simulink model "InductionMotorDrive"  (R2024a)
settings: Solver=FixedStepDiscrete  StartTime=0.0  StopTime=3  RelTol=1e-3  EnableMultiTasking=on
PreLoadFcn:
  | Ts=2e-6;
libraries: spsStairGeneratorLib x3, spsACVoltageSourceLib x1, electricdrivelib x1, sps_lib x1
settings Model: Creator=The MathWorks, Inc.
settings SolverCC: AlgebraicLoopSolver=TrustRegion
settings DataIOCC: SaveFormat=Array  SaveOutput=off  SignalLogging=off  SaveTime=off  ReturnWorkspaceOutputs=off
settings OptimizationCC: LifeSpan=inf
settings DebuggingCC: UnconnectedInputMsg=warning  UnconnectedOutputMsg=warning  UnconnectedLineMsg=warning  SFUnexpectedBacktrackingDiag=warning  SFNoUnconditionalDefaultTransitionDiag=warning  SFExecutionAtInitializationDiag=none  ArithmeticOperatorsInVariantConditions=warning
settings HardwareCC: ProdBitPerSizeT=32  ProdBitPerPtrDiffT=32  ProdWordSize=32  ProdHWDeviceType=Specified
settings ModelReferenceCC: EnableRefExpFcnMdlSchedulingChecks=on
settings SFSimCC: SimUseLocalCustomCode=off  CustomCodeUndefinedFunction=UseInterfaceOnly
settings RTWCC: RTWUseLocalCustomCode=off  GPUComputeCapability=3.5
settings CodeAppCC: StateflowObjectComments=on
settings GRTTargetCC: TargetLangStandard=C89/C90 (ANSI)
settings ConfigComp: CovMetricSettings=dw  CovSaveCumulativeToWorkspaceVar=on  CovSaveSingleToWorkspaceVar=on  CovExternalEMLEnable=off
settings SimscapeCC: SimscapeNormalizeSystem=off  SimscapeNominalValues={1, 'bar'; 1, 'cm^3/s'; 1, 'bar*kg/s'; 1, 'kJ/kg'; 1, 'kW'; }

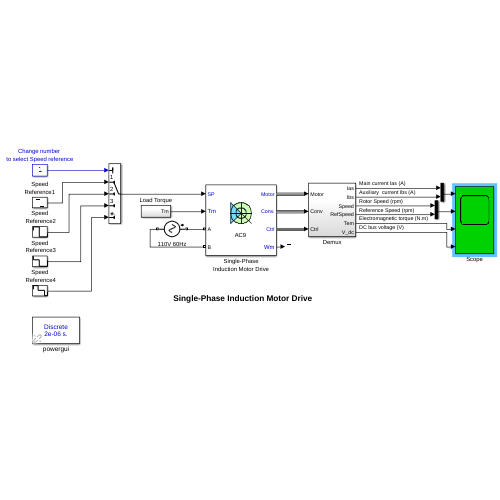
[thumbnail: Simulink's stored preview of the top-level diagram]
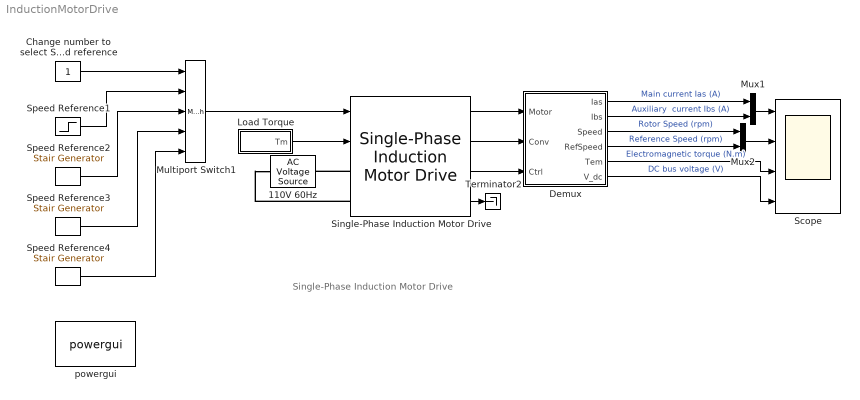
== system InductionMotorDrive ==
  note: Single-Phase Induction Motor Drive
  110V 60Hz : spsACVoltageSourceLib/AC Voltage Source  Amplitude=110*sqrt(2)  Phase=0  Frequency=60  SampleTime=0  Measurements=None  BusType=swing  Pref=10e3  Qref=0  Qmin=-inf  Qmax=+inf
  Change number to select Speed reference : Constant
  Demux : Subsystem
  Load Torque : Subsystem
  Multiport Switch1 : MultiPortSwitch  Inputs=4  InputSameDT=off
  Mux1 : Mux  Inputs=2
  Mux2 : Mux  Inputs=2
  Scope : Scope  NumInputPorts=4
  Single-Phase Induction Motor Drive : electricdrivelib/AC drives/Single-Phase Induction Motor Drive  Pn=0.25*746  Vn=110  fn=60  Rs=2.02  Lls=7.4e-3  Lms=0.1772  Ra=7.14  Lla=8.5e-3  k=1.18  Rr=4.12  Llr=5.6e-3  J=0.0146  Friction=0  p=2  InitialSpeed=0  Rsnubber1=10e3  Csnubber1=20e-9  Ron1=1e-3  Vf1=0.8  cap_bus=39e-4  Rbrake=8  fbrake=4000  activationVoltage=310  shutdownVoltage=300  deviceType=IGBT / Diodes  Ron2=1e-3  Vf2=0  Vfd=0  Rsnubber2=5000  Csnubber2=inf  regulationType=Speed regulation  Tsc=7*20e-6  fc_sc=1000  Acc=1800  Dec=-1800  kp_sc=1  ki_sc=10  Tmin=-4  Tmax=4  in_flux=0.3  nf=0.3  controllerType=FOC  h=0.5  T_bw=0.1  F_bw=0.002  freq_max=20000  Tvect=20e-6  baseSampleTime=2e-06  outputBusMode=Multiple output buses  busLabels=off  MechanicalLoad=Torque Tm  driveType=AC9
  Speed Reference2 : spsStairGeneratorLib/Stair Generator  t=[0 1 1.5 2.2]  e=[500 1000 -500 0]  Ts=Ts
  Speed Reference3 : spsStairGeneratorLib/Stair Generator  t=[0 1 1.5 2.2]  e=[1250 600 -500 500]  Ts=Ts
  Speed Reference4 : spsStairGeneratorLib/Stair Generator  t=[0 1 1.5 2.2 2.5]  e=[500 1000 300 -500 0]  Ts=Ts
  Speed Reference1 : Step  Before=1500  After=750  SampleTime=0
  Terminator2 : Terminator
  powergui : sps_lib/powergui  Priority=2  SimulationMode=Discrete  SampleTime=Ts  frequency=60  Iterations=50  frequencyindice=60  Pbase=100e6  ErrMax=1e-4  UnitsV=kV  UnitsW=MW  buscounter=0  FunctionMessages=off  echomessages=off  EnableUseOfTLC=off  CurrentSourceSwitches=off  DisableSnubberDevices=off  DisableRonSwitches=off  DisableVfSwitches=off  DisplayEquations=off  AutomaticDiscreteSolvers=off  SolverType=Tustin/Backward Euler (TBE)  Interpol=off  ExternalGateDelay=off  methode=off  Ts=0  x0status=blocks  SPID=off  SwTol=0  HookPort=off  NonlinearTolerance=0  nMaxIteration=15  ContinueOnMaxIteration=off  RestoreLinks=warning  ResistiveCurrentMeasurement=off  Frange=[0:2:500]  Ylog=off  Xlog=on  ShowGrid=off  save=off  variable=ZData  structure=0  ZoomFFT=on  StartTime=0.0  cycles=1  DisplayStyle=1  fundamental=60  FreqAxis=off  MaxFrequency=1000  frequencyindicesteady=1  RmsSteady=1  display=off
  wires:
  Single-Phase Induction Motor Drive/4 -> Terminator2/1
  Load Torque/1(Tm) -> Single-Phase Induction Motor Drive/2
  Speed Reference1/1 -> Multiport Switch1/2
  Speed Reference2/1 -> Multiport Switch1/3
  Speed Reference3/1 -> Multiport Switch1/4
  Speed Reference4/1 -> Multiport Switch1/5
  Multiport Switch1/1 -> Single-Phase Induction Motor Drive/1
  Change number to select Speed reference/1 -> Multiport Switch1/1
  Demux/1(Ias) -> Mux1/1  "Main current Ias (A)"
  Demux/2(Ibs) -> Mux1/2  "Auxiliary  current Ibs (A)"
  Demux/3(Speed) -> Mux2/1  "Rotor Speed (rpm)"
  Demux/4(RefSpeed) -> Mux2/2  "Reference Speed (rpm)"
  Mux1/1 -> Scope/1
  Mux2/1 -> Scope/2
  Demux/5(Tem) -> Scope/3  "Electromagnetic torque (N.m)"
  Demux/6(V_dc) -> Scope/4  "DC bus voltage (V)"
  Single-Phase Induction Motor Drive/1 -> Demux/1(Motor)
  Single-Phase Induction Motor Drive/2 -> Demux/2(Conv)
  Single-Phase Induction Motor Drive/3 -> Demux/3(Ctrl)
  connections:
  Single-Phase Induction Motor Drive/LConn1 -- 110V 60Hz/RConn1
  Single-Phase Induction Motor Drive/LConn2 -- 110V 60Hz/LConn1

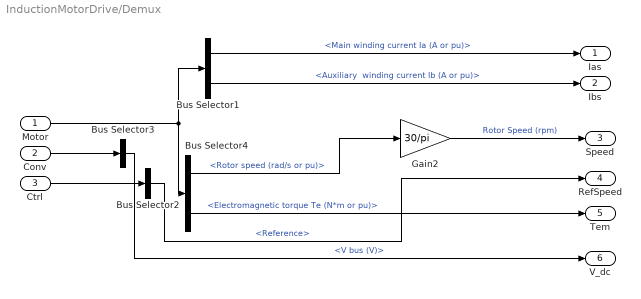
== system InductionMotorDrive/Demux ==
  Motor : Inport
  Conv : Inport  Port=2
  Ctrl : Inport  Port=3
  Bus Selector1 : BusSelector  OutputSignals="Stator measurements.Main winding current Ia (A or pu),Stator measurements.Auxiliary  winding current Ib (A or pu)"
  Bus Selector2 : BusSelector  OutputSignals=Reference
  Bus Selector3 : BusSelector  OutputSignals=V bus (V)
  Bus Selector4 : BusSelector  OutputSignals=Mechanical.Rotor speed (rad/s or pu),Mechanical.Electromagnetic torque Te (N*m or pu)
  Gain2 : Gain  Gain=30/pi  SaturateOnIntegerOverflow=on  OutDataTypeStr=Inherit: Same as input  ParamDataTypeStr=Inherit: Same as input
  Ias : Outport  VectorParamsAs1DForOutWhenUnconnected=off
  Ibs : Outport  Port=2  VectorParamsAs1DForOutWhenUnconnected=off
  Speed : Outport  Port=3  VectorParamsAs1DForOutWhenUnconnected=off
  RefSpeed : Outport  Port=4  VectorParamsAs1DForOutWhenUnconnected=off
  Tem : Outport  Port=5  VectorParamsAs1DForOutWhenUnconnected=off
  V_dc : Outport  Port=6  VectorParamsAs1DForOutWhenUnconnected=off
  wires:
  Bus Selector2/1 -> RefSpeed/1  "<Reference>"
  Bus Selector4/1 -> Gain2/1  "<Rotor speed (rad/s or pu)>"
  Motor/1 -> Bus Selector4/1, Bus Selector1/1
  Conv/1 -> Bus Selector3/1
  Ctrl/1 -> Bus Selector2/1
  Bus Selector3/1 -> V_dc/1  "<V bus (V)>"
  Gain2/1 -> Speed/1  "Rotor Speed (rpm)"
  Bus Selector4/2 -> Tem/1  "<Electromagnetic torque Te (N*m or pu)>"
  Bus Selector1/1 -> Ias/1  "<Main winding current Ia (A or pu)>"
  Bus Selector1/2 -> Ibs/1  "<Auxiliary  winding current Ib (A or pu)>"

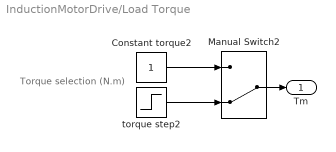
== system InductionMotorDrive/Load Torque ==
  note: Torque selection
      | (N.m)
  Constant torque2 : Constant
  Manual Switch2 : ManualSwitch  CurrentSetting=0
  torque step2 : Step  Time=2  SampleTime=0
  Tm : Outport  VectorParamsAs1DForOutWhenUnconnected=off
  wires:
  torque step2/1 -> Manual Switch2/2
  Constant torque2/1 -> Manual Switch2/1
  Manual Switch2/1 -> Tm/1
